simulink model "BSC_test"  (Simulink 7.4)
settings: Solver=FixedStepDiscrete  StartTime=0.0  StopTime=inf  FixedStep=0.01  RelTol=1e-3
libraries: BSC_lib x1
Description:
  | $Author:Zhao XiangRi$
  | $Date:2015/04/15$
  | $Revision:1.0$
settings Model: Creator=zhaoxiangri  LastModifiedBy=zhaoxiangri
settings DataIOCC: SaveFormat=Structure
settings OptimizationCC: OptimizeModelRefInitCode=on  LifeSpan=1
settings RTWCC: SystemTargetFile=ert.tlc  GenCodeOnly=on  TemplateMakefile=ert_default_tmf  Description=Real-Time Workshop Embedded Coder  ProcessScript=ert_make_rtw_hook
settings CodeAppCC: IgnoreCustomStorageClasses=off
settings ERTTargetCC: MultiwordLength=2048  GenerateSampleERTMain=on  ERTCustomFileTemplate=example_file_process.tlc  ConvertIfToSwitch=off

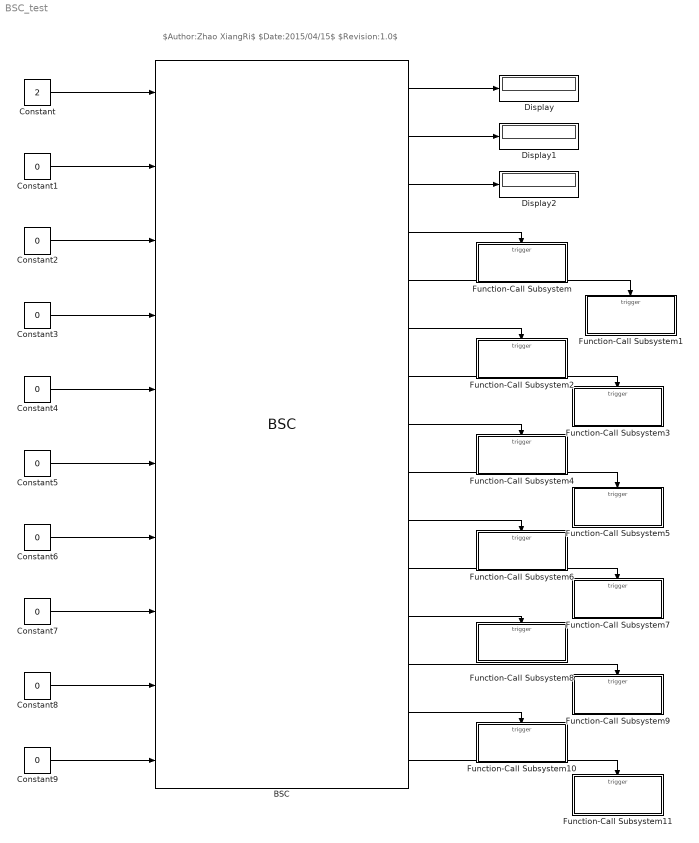
== system BSC_test ==
  note: $Author:Zhao XiangRi$
      | $Date:2015/04/15$
      | $Revision:1.0$
  BSC : BSC_lib/BSC  Description=|  SystemSampleTime=-1
      | $Author:Zhao XiangRi$
      | $Date:2015/03/26$    
      | $Revision:1.0$
  Constant : Constant  Value=2  OutDataTypeMode=uint8  OutDataType=fixdt(1, 16)  OutScaling=2^0  OutDataTypeStr=uint8
  Constant{1..5,9} (6 alike) : Constant  Value=0  OutDataTypeMode=boolean  OutDataType=fixdt(1, 16)  OutScaling=2^0  OutDataTypeStr=boolean
  Constant6 : Constant  Value=0  OutDataTypeMode=uint8  OutDataType=fixdt(1, 16)  OutScaling=2^0  OutDataTypeStr=uint8
  Constant7 : Constant  Value=0  OutDataTypeMode=uint8  OutDataType=fixdt(1, 16)  OutScaling=2^0  OutDataTypeStr=uint8
  Constant8 : Constant  Value=0  OutDataTypeMode=uint8  OutDataType=fixdt(1, 16)  OutScaling=2^0  OutDataTypeStr=uint8
  Display : Display
  Display1 : Display
  Display2 : Display
  Function-Call Subsystem : Subsystem  TreatAsAtomicUnit=on
  Function-Call Subsystem1 : Subsystem  TreatAsAtomicUnit=on
  Function-Call Subsystem10 : Subsystem  TreatAsAtomicUnit=on
  Function-Call Subsystem11 : Subsystem  TreatAsAtomicUnit=on
  Function-Call Subsystem2 : Subsystem  TreatAsAtomicUnit=on
  Function-Call Subsystem3 : Subsystem  TreatAsAtomicUnit=on
  Function-Call Subsystem4 : Subsystem  TreatAsAtomicUnit=on
  Function-Call Subsystem5 : Subsystem  TreatAsAtomicUnit=on
  Function-Call Subsystem6 : Subsystem  TreatAsAtomicUnit=on
  Function-Call Subsystem7 : Subsystem  TreatAsAtomicUnit=on
  Function-Call Subsystem8 : Subsystem  TreatAsAtomicUnit=on
  Function-Call Subsystem9 : Subsystem  TreatAsAtomicUnit=on
  wires:
  BSC/1 -> Display/1
  BSC/2 -> Display1/1
  Constant/1 -> BSC/1
  Constant1/1 -> BSC/2
  Constant2/1 -> BSC/3
  Constant3/1 -> BSC/4
  Constant4/1 -> BSC/5
  Constant5/1 -> BSC/6
  Constant6/1 -> BSC/7
  Constant7/1 -> BSC/8
  Constant8/1 -> BSC/9
  Constant9/1 -> BSC/10
  BSC/4 -> Function-Call Subsystem/Trigger
  BSC/5 -> Function-Call Subsystem1/Trigger
  BSC/6 -> Function-Call Subsystem2/Trigger
  BSC/7 -> Function-Call Subsystem3/Trigger
  BSC/8 -> Function-Call Subsystem4/Trigger
  BSC/9 -> Function-Call Subsystem5/Trigger
  BSC/10 -> Function-Call Subsystem6/Trigger
  BSC/11 -> Function-Call Subsystem7/Trigger
  BSC/12 -> Function-Call Subsystem8/Trigger
  BSC/13 -> Function-Call Subsystem9/Trigger
  BSC/14 -> Function-Call Subsystem10/Trigger
  BSC/15 -> Function-Call Subsystem11/Trigger
  BSC/3 -> Display2/1

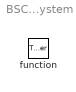
== system BSC_test/Function-Call Subsystem ==
  function : TriggerPort  TriggerType=function-call

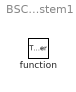
== system BSC_test/Function-Call Subsystem1 ==
  function : TriggerPort  TriggerType=function-call

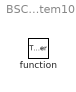
== system BSC_test/Function-Call Subsystem10 ==
  function : TriggerPort  TriggerType=function-call

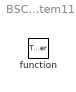
== system BSC_test/Function-Call Subsystem11 ==
  function : TriggerPort  TriggerType=function-call

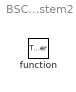
== system BSC_test/Function-Call Subsystem2 ==
  function : TriggerPort  TriggerType=function-call

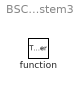
== system BSC_test/Function-Call Subsystem3 ==
  function : TriggerPort  TriggerType=function-call

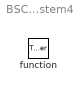
== system BSC_test/Function-Call Subsystem4 ==
  function : TriggerPort  TriggerType=function-call

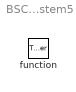
== system BSC_test/Function-Call Subsystem5 ==
  function : TriggerPort  TriggerType=function-call

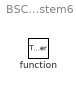
== system BSC_test/Function-Call Subsystem6 ==
  function : TriggerPort  TriggerType=function-call

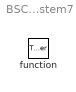
== system BSC_test/Function-Call Subsystem7 ==
  function : TriggerPort  TriggerType=function-call

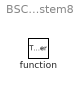
== system BSC_test/Function-Call Subsystem8 ==
  function : TriggerPort  TriggerType=function-call

== system BSC_test/Function-Call Subsystem9 ==
  function : TriggerPort  TriggerType=function-call
